simulink model "PatientModelOL_DL (1)"  (R2020a)
settings: Solver=VariableStepAuto  StartTime=0.0  StopTime=24*60  RelTol=1e-3
model workspace (MAT data in the model file):
  Cden = Simulink.Parameter
  Cden.Value = [0 0 0 0 0 0 0 0 0 1]
  Cden.DataType = 'auto'
  Cden.Dimensions = [1 10]
  Cnum = Simulink.Parameter
  Cnum.Value = [0 0 0 0 0 0 0 0 0 1]
  Cnum.DataType = 'auto'
  Cnum.Dimensions = [1 10]
  params = Simulink.Parameter
  params.Value = [1541.03560355 12.1141885316 0.00903725375345 138.323022044 0 0.00350657503829 0 19.3120138461 97.2866168168 161.047932197 158.685488242 0 0 0 0 0 0 0 0 0]
  params.DataType = 'auto'
  params.Dimensions = [1 20]
settings Model: Creator=vjoukov  LastModifiedBy=nafisfuad
settings DataIOCC: ReturnWorkspaceOutputs=off
settings DebuggingCC: ArithmeticOperatorsInVariantConditions=warning
settings SFSimCC: SimUseLocalCustomCode=off  CustomCodeUndefinedFunction=UseInterfaceOnly
settings RTWCC: RTWUseLocalCustomCode=off

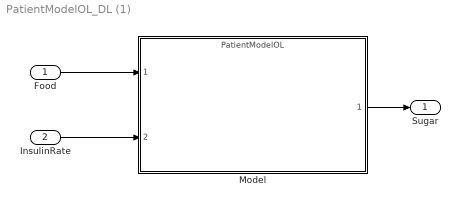
== system PatientModelOL_DL (1) ==
  Food : Inport
  InsulinRate : Inport  Port=2
  Model : ModelReference  ModelNameDialog=PatientModelOL.slxp  ParameterArgumentNames=params  ParameterArgumentValues=params  UsingDefaultArgumentValue=0  ModelReferenceVersion=1.387  CopyOfModelProtected=on
  Sugar : Outport  VectorParamsAs1DForOutWhenUnconnected=off
  wires:
  Food/1 -> Model/1
  InsulinRate/1 -> Model/2
  Model/1 -> Sugar/1
